simulink model "BrakingSystem"  (Simulink 7.8)
settings: Solver=ode45  StartTime=0.0  StopTime=10.0  RelTol=1e-3
settings Model: Creator=ah875096  LastModifiedBy=Arne Haber

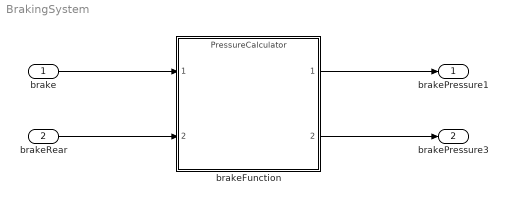
== system BrakingSystem ==
  brake : Inport
  brakeRear : Inport  Port=2
  brakeFunction : ModelReference  ModelNameDialog=PressureCalculator  SimulationMode=Normal  ModelReferenceVersion=1.7  CopyOfModelName=PressureCalculator  DefaultDataLogging=on
  brakePressure1 : Outport
  brakePressure3 : Outport  Port=2
  wires:
  brake/1 -> brakeFunction/1
  brakeFunction/1 -> brakePressure1/1
  brakeFunction/2 -> brakePressure3/1
  brakeRear/1 -> brakeFunction/2
